simulink model "EvPowertrainController2EM_r3_23a"  (R2023a)
settings: configuration reference "VehicleFixed10ms" (kept outside this file)
model workspace (MAT data in the model file):
  CtrlVcuAccelPdlBpts = [0 0.8 1]
  CtrlVcuBattPnlty = 10000000
  CtrlVcuBattSOCBpts = [0 20 60 80 100]
  CtrlVcuCnstrntPnltyFctr = 10000000
  CtrlVcuEMPnlty = 100
  CtrlVcuEMTrqSplitGrid = 200
  CtrlVcuFallRate = -500
  CtrlVcuMaxAccelG = 1
  CtrlVcuMaxDecelG = -1.5
  CtrlVcuPwrDeltaPnlty = 50
  CtrlVcuPwrRatePnlty = [25 25 100]
  CtrlVcuRiseRate = 500
  CtrlVcuRoadMuEst = 0.8
  CtrlVcuSftyFctr = 0.9
  CtrlVcuTracPwrErrPnlty = 25
  CtrlVcuTrqVecBrkThresh = 0.01
  CtrlVcuTrqVecIGain = 0
  CtrlVcuTrqVecMinTrq = 25
  CtrlVcuTrqVecPGain = -2000
  CtrlVcuTrqVecSteerThresh = 0.349065850399
  CtrlVcuTrqVecVelThresh = 2.5
  N_P0 = 3
settings Model: DataDictionary=VirtualVehicleTemplate.sldd  ModifiedByFormat=The MathWorks, Inc.  Creator=The MathWorks, Inc.  LastModifiedBy=The MathWorks, Inc.
settings ConfigSetRef: SourceName=VehicleFixed10ms

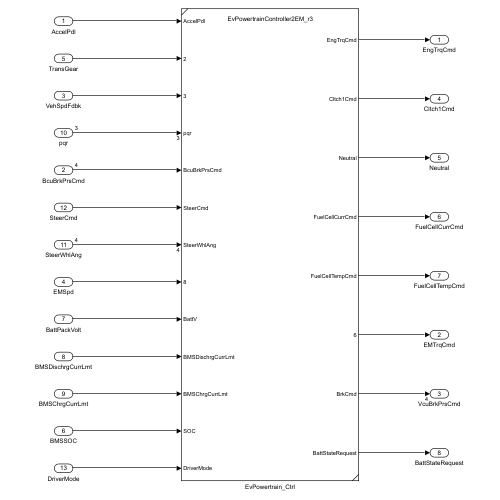
[thumbnail: Simulink's stored preview of the top-level diagram]
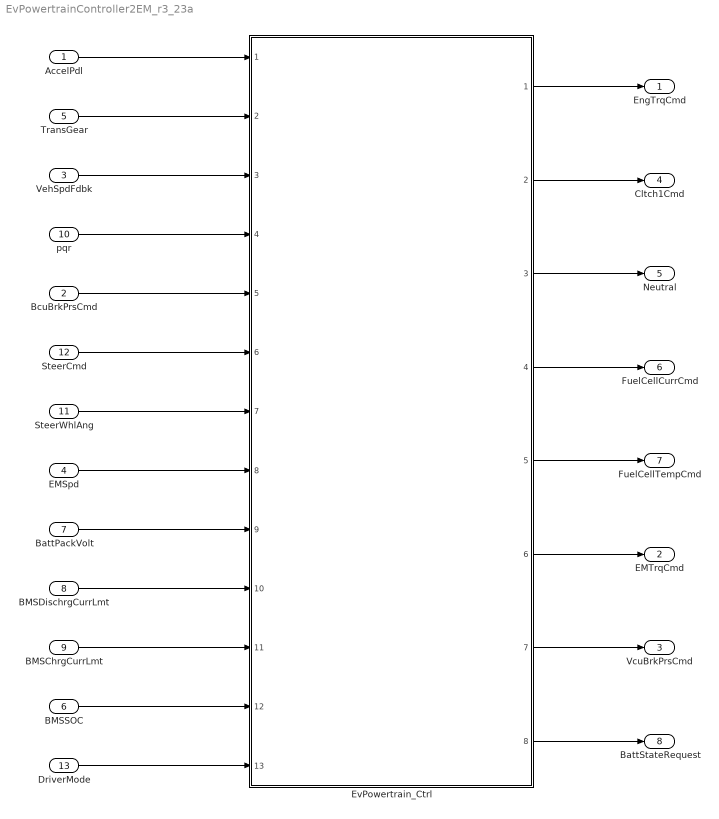
== system EvPowertrainController2EM_r3_23a ==
  AccelPdl : Inport  OutDataTypeStr=double  PortDimensions=1
  BcuBrkPrsCmd : Inport  Port=2  OutDataTypeStr=double  PortDimensions=4
  VehSpdFdbk : Inport  Port=3  OutDataTypeStr=double  PortDimensions=1
  EMSpd : Inport  Port=4  OutDataTypeStr=double
  TransGear : Inport  Port=5  OutDataTypeStr=double  PortDimensions=1
  BMSSOC : Inport  Port=6
  BattPackVolt : Inport  Port=7
  BMSDischrgCurrLmt : Inport  Port=8
  BMSChrgCurrLmt : Inport  Port=9
  pqr : Inport  Port=10  PortDimensions=3
  SteerWhlAng : Inport  Port=11  PortDimensions=4
  SteerCmd : Inport  Port=12
  DriverMode : Inport  Port=13  OutDataTypeStr=Enum: DriverMode
  EvPowertrain_Ctrl : Subsystem  ReferencedSubsystem=EvPowertrainController2EM_r3
  EngTrqCmd : Outport  OutDataTypeStr=double  PortDimensions=1  VectorParamsAs1DForOutWhenUnconnected=off
  EMTrqCmd : Outport  Port=2  OutDataTypeStr=double  VectorParamsAs1DForOutWhenUnconnected=off
  VcuBrkPrsCmd : Outport  Port=3  OutDataTypeStr=double  PortDimensions=4  VectorParamsAs1DForOutWhenUnconnected=off
  Cltch1Cmd : Outport  Port=4  OutDataTypeStr=double  PortDimensions=1  VectorParamsAs1DForOutWhenUnconnected=off
  Neutral : Outport  Port=5  OutDataTypeStr=double  PortDimensions=1  VectorParamsAs1DForOutWhenUnconnected=off
  FuelCellCurrCmd : Outport  Port=6  OutDataTypeStr=double  PortDimensions=1
  FuelCellTempCmd : Outport  Port=7  OutDataTypeStr=double  PortDimensions=1
  BattStateRequest : Outport  Port=8  OutDataTypeStr=Enum: SRE  PortDimensions=1
  wires:
  EvPowertrain_Ctrl/6 -> EMTrqCmd/1
  BMSChrgCurrLmt/1 -> EvPowertrain_Ctrl/11
  SteerWhlAng/1 -> EvPowertrain_Ctrl/7
  SteerCmd/1 -> EvPowertrain_Ctrl/6
  AccelPdl/1 -> EvPowertrain_Ctrl/1
  TransGear/1 -> EvPowertrain_Ctrl/2
  EMSpd/1 -> EvPowertrain_Ctrl/8
  BattPackVolt/1 -> EvPowertrain_Ctrl/9
  pqr/1 -> EvPowertrain_Ctrl/4
  BMSDischrgCurrLmt/1 -> EvPowertrain_Ctrl/10
  VehSpdFdbk/1 -> EvPowertrain_Ctrl/3
  BcuBrkPrsCmd/1 -> EvPowertrain_Ctrl/5
  BMSSOC/1 -> EvPowertrain_Ctrl/12
  DriverMode/1 -> EvPowertrain_Ctrl/13
  EvPowertrain_Ctrl/1 -> EngTrqCmd/1
  EvPowertrain_Ctrl/2 -> Cltch1Cmd/1
  EvPowertrain_Ctrl/3 -> Neutral/1
  EvPowertrain_Ctrl/4 -> FuelCellCurrCmd/1
  EvPowertrain_Ctrl/5 -> FuelCellTempCmd/1
  EvPowertrain_Ctrl/8 -> BattStateRequest/1
  EvPowertrain_Ctrl/7 -> VcuBrkPrsCmd/1
